simulink model "Sum1"  (R2020b)
settings: Solver=VariableStepAuto  StartTime=0.0  StopTime=10.0  RelTol=1e-3
undefined symbols (not defined in the file): b, k1, k12, m1, m2
settings Model: Creator=Aradhana desai  LastModifiedBy=Aradhana desai

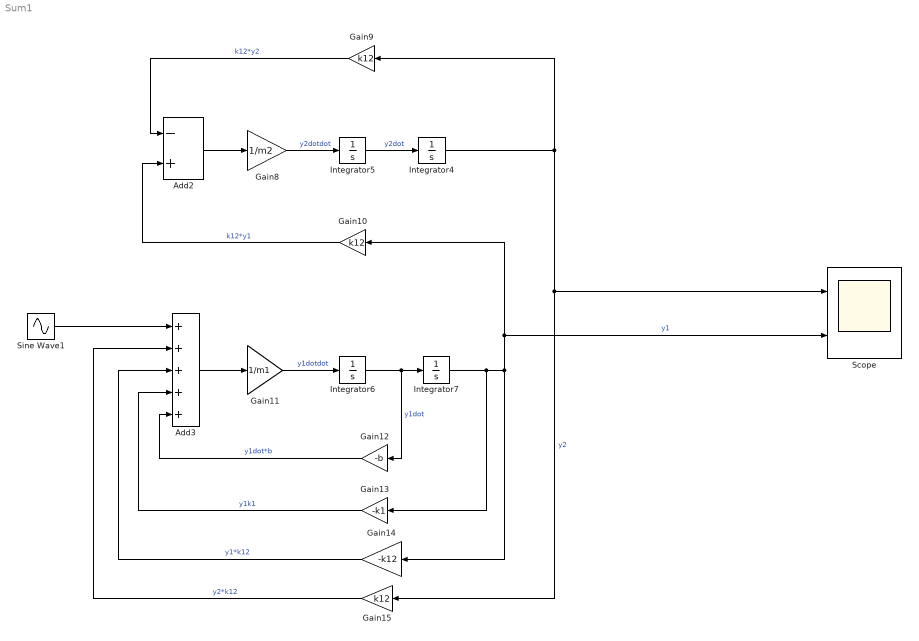
== system Sum1 ==
  Add2 : Sum  Inputs=-+
  Add3 : Sum  Inputs=+++++
  Gain10 : Gain  Gain=k12
  Gain11 : Gain  Gain=1/m1
  Gain12 : Gain  Gain=-b
  Gain13 : Gain  Gain=-k1
  Gain14 : Gain  Gain=-k12
  Gain15 : Gain  Gain=k12
  Gain8 : Gain  Gain=1/m2
  Gain9 : Gain  Gain=k12
  Integrator{4..7} (4 alike) : Integrator
  Scope : Scope  NumInputPorts=2
  Sine Wave1 : Sin  Amplitude=2  Frequency=10  SampleTime=0
  wires:
  Gain13/1 -> Add3/4  "y1k1"
  Add2/1 -> Gain8/1
  Sine Wave1/1 -> Add3/1
  Gain15/1 -> Add3/2  "y2*k12"
  Gain14/1 -> Add3/3  "y1*k12"
  Gain11/1 -> Integrator6/1  "y1dotdot"
  Integrator6/1 -> Gain12/1, Integrator7/1  "y1dot"
  Gain8/1 -> Integrator5/1  "y2dotdot"
  Integrator7/1 -> Gain13/1, Gain10/1, Scope/2, Gain14/1  "y1"
  Add3/1 -> Gain11/1
  Gain9/1 -> Add2/1  "k12*y2"
  Gain10/1 -> Add2/2  "k12*y1"
  Integrator5/1 -> Integrator4/1  "y2dot"
  Gain12/1 -> Add3/5  "y1dot*b"
  Integrator4/1 -> Scope/1, Gain15/1, Gain9/1  "y2"
